simulink model "dsPIC33CDVL64MC106_SMO"  (R2023b)
settings: Solver=FixedStepDiscrete  StartTime=0.0  StopTime=15  FixedStep=.00005  RelTol=1e-3
PostLoadFcn:
  | dsPIC33CDVL64MC106_SMO_data;
InitFcn:
  | dsPIC33CDVL64MC106_SMO_data;
values from neighbouring files (symbols this model uses):
  i_base = inverter.ISenseMax    [dsPIC33CDVL64MC106_SMO_data.m]
  Iq_Ref_openLoop = 0.95    [dsPIC33CDVL64MC106_SMO_data.m]
  PI_params = mcb.internal.SetControllerParameters(pmsm,inverter,PU_System,T_pwm,Ts,Ts_speed)    [dsPIC33CDVL64MC106_SMO_data.m]
  PU_System = mcb_SetPUSystem(pmsm,inverter)    [dsPIC33CDVL64MC106_SMO_data.m]
  PWM_frequency = 20e3    (= 20000)    [dsPIC33CDVL64MC106_SMO_data.m]
  Speed_Ref_openLoop = 700    [dsPIC33CDVL64MC106_SMO_data.m]
  Ts = T_pwm    (= 5e-05)    [dsPIC33CDVL64MC106_SMO_data.m]
  Ts_speed = 30*Ts    (= 0.0015)    [dsPIC33CDVL64MC106_SMO_data.m]
  Vs_max_pu = V_max/PU_System.V_base    [dsPIC33CDVL64MC106_SMO_data.m]
undefined symbols (not defined in the file or in its folder): A4, B0, C10, C11, C12, C4, C7, C8, C9, D10, DiscIntNeverNeededParam, internal, inverter, Max, MaxPer, ms, NumBits1, NumBits2, P20, P32, P52, P55, P56, P57, P58, P59, P60, P74, Pin, pmsm, PWM1max, Resol, s, us
libraries: simulink x32, MCHP_Blockset x22, mcbcontrolslib x9, slpidlib x3, mcbplantlib x1, autolibpmsmexterior x1
(part 1 of 4)
settings Model: Creator=M91449  LastModifiedBy=I52209
settings SolverCC: AlgebraicLoopSolver=TrustRegion
settings DataIOCC: LimitDataPoints=on  ReturnWorkspaceOutputs=off
settings OptimizationCC: DefaultParameterBehavior=Inlined  InlineInvariantSignals=on  ReuseModelBlockBuffer=off  LifeSpan=1  EfficientTunableParamExpr=on
settings DebuggingCC: MultiTaskDSMMsg=none  ParameterOverflowMsg=none  UnconnectedInputMsg=warning  UnconnectedOutputMsg=warning  UnconnectedLineMsg=warning  SFUnexpectedBacktrackingDiag=warning  SFNoUnconditionalDefaultTransitionDiag=warning  SFExecutionAtInitializationDiag=none  ArithmeticOperatorsInVariantConditions=warning
settings HardwareCC: ProdBitPerInt=16  ProdBitPerPointer=16  ProdBitPerSizeT=16  ProdBitPerPtrDiffT=16  ProdLargestAtomicInteger=Integer  ProdLargestAtomicFloat=None  ProdWordSize=16  ProdHWDeviceType=Generic->Custom
settings ModelReferenceCC: EnableRefExpFcnMdlSchedulingChecks=on  ModelReferenceNumInstancesAllowed=Single  PropagateSignalLabelsOutOfModel=off
settings SFSimCC: SimUseLocalCustomCode=off  MATLABDynamicMemAlloc=off  CustomCodeUndefinedFunction=UseInterfaceOnly
settings RTWCC: Description=Microchip Embedded Target PIC24 dsPIC30 dsPIC33 (real-time)  SystemTargetFile=MCHP_dsPIC_stf.tlc  TemplateMakefile=MCHP_dsPIC.tmf  RTWUseLocalCustomCode=off  IncludeHyperlinkInReport=on  GenerateCodeMetricsReport=on  DLArmComputeVersion=19.05
settings RTWCC: CustomSourceCode=|
  | void port_pull_up_enable(void)
  | {
  |     _CNPUC12 = 1;
  |     _CNPUD1 = 1;
  | }
settings CodeAppCC: IgnoreCustomStorageClasses=off  MaxIdLength=255  StateflowObjectComments=on
settings STFCustomTargetCC: TargetLibSuffix=_lib.a  TargetLangStandard=C89/C90 (ANSI)  CodeReplacementLibrary=Microchip Code Replacement Library for dsPIC  CombineOutputUpdateFcns=on  ERTCustomFileBanners=on  SupportContinuousTime=off  RemoveResetFunc=on  MATLABClassNameForMDSCustomization=Simulink.SoftwareTarget.ERTCustomization  SystemTargetFile=MCHP_dsPIC_stf.tlc
settings ERTTargetCC: TargetLibSuffix=_lib.a  CodeReplacementLibrary=Microchip Code Replacement Library for dsPIC  MultiwordLength=2048  ParMdlRefBuildCompliant=off  CompOptLevelCompliant=off  ConcurrentExecutionCompliant=off  SupportNonInlinedSFcns=on  ModelStepFunctionPrototypeControlCompliant=off  CPPClassGenCompliant=off  UseToolchainInfoCompliant=off  InlinedParameterPlacement=NonHierarchical  ERTSrcFileBannerTemplate=MCHP_dsPIC_code_template.cgt  ERTHdrFileBannerTemplate=MCHP_dsPIC_code_template.cgt  ERTDataSrcFileTemplate=MCHP_dsPIC_code_template.cgt  ERTDataHdrFileTemplate=MCHP_dsPIC_code_template.cgt  ERTCustomFileTemplate=MCHP_main.tlc  ConvertIfToSwitch=off  SuppressUnreachableDefaultCases=off
settings ConfigComp: CovMetricSettings=dw  CovSaveCumulativeToWorkspaceVar=on  CovSaveSingleToWorkspaceVar=on  CovExternalEMLEnable=off

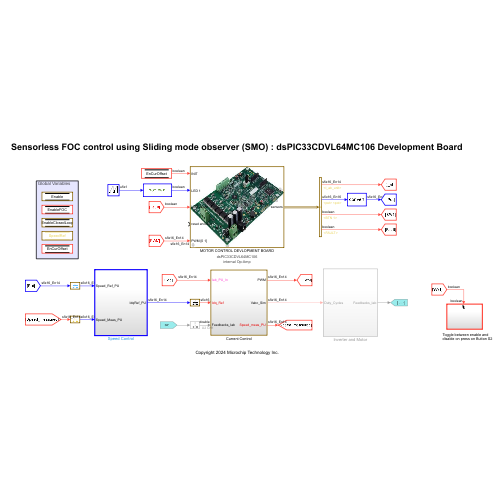
[thumbnail: Simulink's stored preview of the top-level diagram]
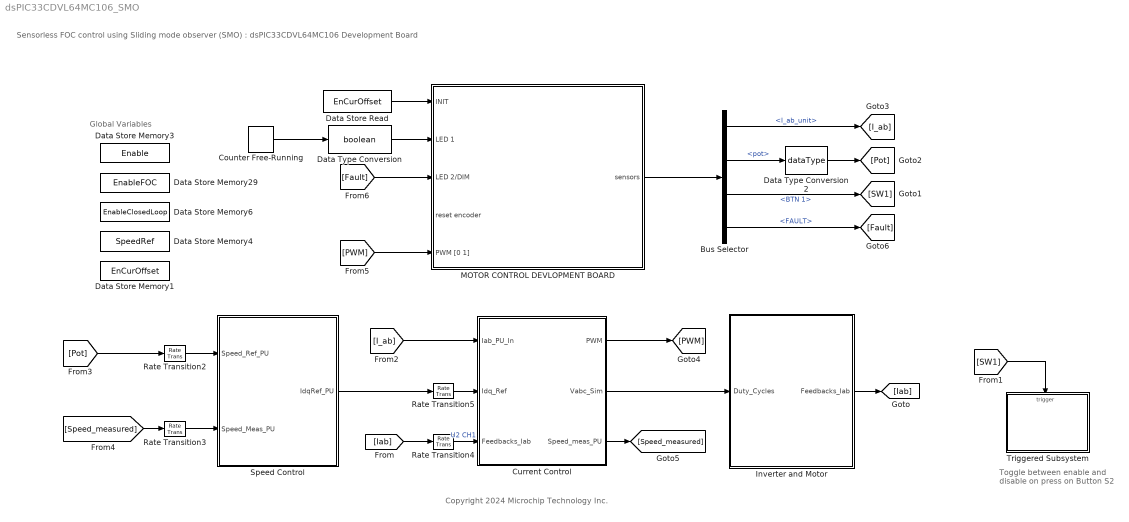
== system dsPIC33CDVL64MC106_SMO ==
  note: Global Variables
  note: Copyright 2024 Microchip Technology Inc.
  note: Sensorless FOC control using Sliding mode observer (SMO) : dsPIC33CDVL64MC106 Development Board
  note: Toggle between enable and disable on press on Button S2
  Bus Selector : BusSelector  OutputSignals=ADC_unit.I_ab_unit,ADC.pot,BTN.BTN 1,Board specific.FAULT
  Counter Free-Running : simulink/Sources/Counter Free-Running  NumBits=1  tsamp=0.5
  Current Control : Subsystem
  Data Store Memory1 : DataStoreMemory  DataStoreName=EnCurOffset  ShowAdditionalParam=off  OutDataTypeStr=boolean
  Data Store Memory29 : DataStoreMemory  DataStoreName=EnableFOC  ShowAdditionalParam=off  OutDataTypeStr=boolean
  Data Store Memory3 : DataStoreMemory  DataStoreName=Enable  ShowAdditionalParam=off  OutDataTypeStr=boolean
  Data Store Memory4 : DataStoreMemory  DataStoreName=SpeedRef  ShowAdditionalParam=off  OutDataTypeStr=dataType
  Data Store Memory6 : DataStoreMemory  DataStoreName=EnableClosedLoop  ShowAdditionalParam=off  OutDataTypeStr=boolean
  Data Store Read : DataStoreRead  DataStoreName=EnCurOffset  IndexOptions=Index vector (dialog)  Indices=1  OutputSizes=1
  Data Type Conversion : DataTypeConversion  OutDataTypeStr=boolean  SaturateOnIntegerOverflow=off  RndMeth=Floor
  Data Type Conversion2 : DataTypeConversion  OutDataTypeStr=dataType  RndMeth=Simplest  SaturateOnIntegerOverflow=off
  Inverter and Motor : Subsystem
  MOTOR CONTROL DEVLOPMENT BOARD : Subsystem  mask(MCLV-48V-300W - dsPIC33CK64MC105 MC DIM using internal Op-Amp){TargetedChip=dsPIC33CDVL64MC106, boardVariants=internal Op-Amp, n=pmsm.p, QEIResolution=1000, QEI_Reset=on logical input (software), QEI_Offset_settings=0, QEIOffset=0}
      mask prompts: TargetedChip "Embedded Chip"; boardVariants "board variants"; n "Motor poles pairs"; QEIResolution "Optical encoder resolution per mechanical rotation (lines)"; QEI_Reset "Optical encoder reset"; QEI_Offset_settings "Optical encoder offset (mechanical in rad)"; QEIOffset "Optical encoder offset (mechanical in rad)"
      mask help:
      | Template for motor control algorithm. Open subsystem (ctrl-u) for further customisation.
      |
      | Block bus output provices:
      |   - Current phase ia & ib, DC bus and potentiometer position
      |   - Buttons (0 when pressed, 1 for Btn 3 unconnected)
      |   - QEI position and velocity
      |   - MCU load and overload
      |
      | Block inputs:
      |   - INIT signal average the current phase ia and ib to be removed
      |   - LEDs
      |   - Reset encoder allows to align the motor while reseting the encoder
      |   - PWM normalized duty cycle value
      |
      | Model 50us base rate (20kHz) is synchronized with ADC conversion which is synchronized with the 50us PWM periods
      mask init:
      | MCHP_MASTERLINK = find_system(gcb,'FollowLinks','on','LookUnderMasks','all','ReferenceBlock','MCHP_Blockset/System Configuration/Microchip Master');
      | if numel(MCHP_MASTERLINK) >= 1
      |     TargetedChip_value = get_param(gcb,'TargetedChip');
      |     TargetedChip_value = TargetedChip_value(6:end); % remove dsPIC
      |     if ~strcmp(get_param(MCHP_MASTERLINK{1},'PICREF'),TargetedChip_value)
      |         set_param(MCHP_MASTERLINK{1},'PICREF',TargetedChip_value);        
      |     end
      | end
      | 
      | BlksQEI = find_system(gcb,'FollowLinks','on','LookUnderMasks','all','ReferenceBlock','MCHP_Blockset/QEI/QEI');
      | QEI_Reset = get_param(gcb,'QEI_Reset');
      | if numel(BlksQEI) >= 1
      |     switch QEI_Reset
      |         case 'on index signal'
      |             set_param(BlksQEI{1},'PIMOD_mode','RESET position on each INDEX event');
      |         case 'on logical input (software)'        
      |             set_param(BlksQEI{1},'PIMOD_mode','position is cyclique between user defined boundaries'); 
      |         case 'custom setting'
      |             % do nothing 
      |     end
      | end % if
      | 
      |     BlksOpAmp = find_system(gcb,'FollowLinks','on','IncludeCommented','on','LookUnderMasks','all','ReferenceBlock','MCHP_Blockset/Analog IO/Op-Amp');
      |     if numel(BlksOpAmp) >= 1
      |         boardVariants = get_param(gcb,'boardVariants');
      |         switch boardVariants
      |             case 'internal Op-Amp'
      |                 if ~strcmp(get_param(BlksOpAmp{1},'Commented'),'off')
      |                     set_param(BlksOpAmp{1},'Commented','off');
      |                 end
      |             case 'external Op-Amp'
      |                 if ~strcmp(get_param(BlksOpAmp{1},'Commented'),'on')
      |                     set_param(BlksOpAmp{1},'Commented','on');
      |                 end
      |         end
      |     end % if
      settings: AttributesFormatString=|
      | %<TargetedChip>
      | %<boardVariants>
      mask TypeOptions TargetedChip: dsPIC33CDVL64MC106 | dsPIC33CDV64MC106
      mask TypeOptions boardVariants: internal Op-Amp | external Op-Amp
      mask TypeOptions QEI_Reset: on index signal | on logical input (software) | custom setting
      mask Callback QEI_Reset:
      | QEI_Reset = get_param(gcb,'QEI_Reset');
      | switch QEI_Reset
      |     case 'on index signal'
      |         QEIOffset = MCHP_Fun.Evalin('base','QEIOffset');
      |         set_param(gcb,'QEIOffset',num2str(QEIOffset));
      |         set_param(gcb,'MaskVisibilities',{'on';'on';'on';'on';'on';'on';'off'});
      |     case 'on logical input (software)'
      |         set_param(gcb,'QEIOffset','0');
      |         set_param(gcb,'MaskVisibilities',{'on';'on';'on';'on';'on';'off';'off'});
      |     case 'custom setting'
      |         set_param(gcb,'MaskVisibilities',{'on';'on';'on';'on';'on';'on';'off'});
      |         % do nothing
      | end
      mask DialogControl n Tooltip: Number of pole pairs of the motor
      mask DialogControl QEIResolution Tooltip: encoder resolution per mechanical rotation
      mask DialogControl QEI_Reset Tooltip: enable encoder index signal if available. Otherwise align motor by applying a tension and set the rst input to 1
      mask DialogControl QEI_Offset_settings Tooltip: offset angle between encoder index and motor winding reference axis applied on theta_m and theta_e
      mask Display: image('MCHP_i_Board_MotorControlDevBoard_33CDV64MC106.jpg');
  Rate Transition{2..5} (4 alike) : RateTransition  Deterministic=off
  Speed Control : Subsystem  TreatAsAtomicUnit=on  SystemSampleTime=Ts_speed
  Triggered Subsystem : Subsystem  TreatAsAtomicUnit=on
  wires:
  MOTOR CONTROL DEVLOPMENT BOARD/1(sensors) -> Bus Selector/1
  [Iab] -> Rate Transition4/1
  Rate Transition3/1 -> Speed Control/2(Speed_Meas_PU)
  Data Type Conversion/1 -> MOTOR CONTROL DEVLOPMENT BOARD/2(LED 1)
  Rate Transition5/1 -> Current Control/2(Idq_Ref)
  [Fault] -> MOTOR CONTROL DEVLOPMENT BOARD/3(LED 2/DIM)
  [Speed_measured] -> Rate Transition3/1
  Bus Selector/1 -> [I_ab]  "<I_ab_unit>"
  Current Control/3(Speed_meas_PU) -> [Speed_measured]
  [Pot] -> Rate Transition2/1
  [PWM] -> MOTOR CONTROL DEVLOPMENT BOARD/5(PWM [0 1])
  [I_ab] -> Current Control/1(Iab_PU_In)
  Rate Transition2/1 -> Speed Control/1(Speed_Ref_PU)
  Current Control/1(PWM) -> [PWM]
  Counter Free-Running/1 -> Data Type Conversion/1
  Data Type Conversion2/1 -> [Pot]
  Bus Selector/2 -> Data Type Conversion2/1  "<pot>"
  Rate Transition4/1 -> Current Control/3(Feedbacks_Iab)  "U2 CH1"
  [SW1] -> Triggered Subsystem/Trigger
  Bus Selector/3 -> [SW1]  "<BTN 1>"
  Inverter and Motor/1(Feedbacks_Iab) -> [Iab]
  Speed Control/1(IdqRef_PU) -> Rate Transition5/1
  Current Control/2(Vabc_Sim) -> Inverter and Motor/1(Duty_Cycles)
  Bus Selector/4 -> [Fault]  "<FAULT>"
  Data Store Read/1 -> MOTOR CONTROL DEVLOPMENT BOARD/1(INIT)

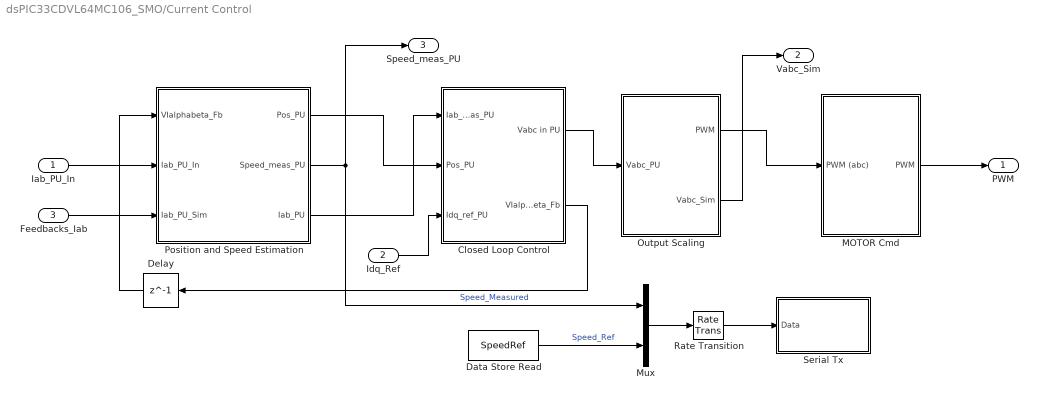
== system dsPIC33CDVL64MC106_SMO/Current Control ==
  Iab_PU_In : Inport
  Idq_Ref : Inport  Port=2
  Feedbacks_Iab : Inport  Port=3
  Closed Loop Control : Subsystem
  Data Store Read : DataStoreRead  DataStoreName=SpeedRef  IndexOptions=Index vector (dialog)  Indices=1  OutputSizes=1
  Delay : Delay  DelayLength=1
  MOTOR Cmd : Subsystem
  Mux : Mux  Inputs=2
  Output Scaling : Subsystem
  Position and Speed Estimation : Subsystem
  Rate Transition : RateTransition  Integrity=off  Deterministic=off  OutPortSampleTime=Ts*100
  Serial Tx : Subsystem
  PWM : Outport
  Vabc_Sim : Outport  Port=2
  Speed_meas_PU : Outport  Port=3
  wires:
  Output Scaling/1(PWM) -> MOTOR Cmd/1(PWM (abc))
  Closed Loop Control/1(Vabc in PU) -> Output Scaling/1(Vabc_PU)
  MOTOR Cmd/1(PWM) -> PWM/1
  Iab_PU_In/1 -> Position and Speed Estimation/2(Iab_PU_In)
  Closed Loop Control/2(VIalphabeta_Fb) -> Delay/1
  Delay/1 -> Position and Speed Estimation/1(VIalphabeta_Fb)
  Idq_Ref/1 -> Closed Loop Control/3(Idq_ref_PU)
  Position and Speed Estimation/1(Pos_PU) -> Closed Loop Control/2(Pos_PU)
  Position and Speed Estimation/3(Iab_PU) -> Closed Loop Control/1(Iab_meas_PU)
  Feedbacks_Iab/1 -> Position and Speed Estimation/3(Iab_PU_Sim)
  Output Scaling/2(Vabc_Sim) -> Vabc_Sim/1
  Data Store Read/1 -> Mux/2  "Speed_Ref"
  Rate Transition/1 -> Serial Tx/1(Data)
  Position and Speed Estimation/2(Speed_meas_PU) -> Mux/1, Speed_meas_PU/1  "Speed_Measured"
  Mux/1 -> Rate Transition/1

== system dsPIC33CDVL64MC106_SMO/Inverter and Motor ==
  Duty_Cycles : Inport
  Codegeneration : Subsystem
  Simulation : Subsystem
  Variant Sink : VariantSink
  Variant Source : VariantSource
  Feedbacks_Iab : Outport  VectorParamsAs1DForOutWhenUnconnected=off
  wires:
  Codegeneration/1(Feedbacks_Iab) -> Variant Source/1
  Variant Sink/1 -> Codegeneration/1(Duty_Cycles)
  Simulation/1(Feedbacks_Iab) -> Variant Source/2
  Variant Sink/2 -> Simulation/1(Duty_Cycles)
  Variant Source/1 -> Feedbacks_Iab/1
  Duty_Cycles/1 -> Variant Sink/1
